simulink model "wing_landing_gear"  (R2015a)
settings: Solver=ode45  StartTime=0  StopTime=10  RelTol=1e-4  AbsTol=1e-4
model workspace (MAT data in the model file):
  grey = [0.5 0.5 0.5]
  lgrey = [0.7 0.7 0.7]
  dgrey = [0.3 0.3 0.3]
  ddgrey = [0.15 0.15 0.15]
  rho_alum = 2700
undefined symbols (not defined in the file): sigbuilder_block, X, Y, Z
libraries: sm_lib x59, sm_wing_landing_gear_lib x45, nesl_utility x7, simulink x2
(part 2 of 3)

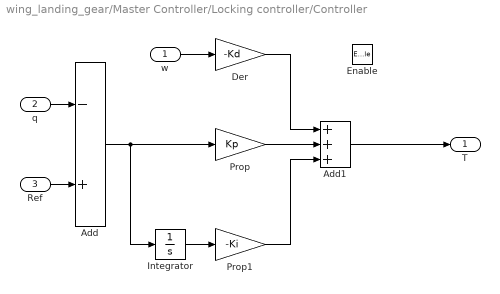
== system wing_landing_gear/Master Controller/Locking controller/Controller ==
  w : Inport
  q : Inport  Port=2
  Ref : Inport  Port=3
  Enable : EnablePort  StatesWhenEnabling=reset
  Add : Sum  Inputs=-+
  Add1 : Sum  Inputs=+++
  Der : Gain  Gain=-Kd
  Integrator : Integrator
  Prop : Gain  Gain=Kp
  Prop1 : Gain  Gain=-Ki
  T : Outport
  wires:
  Ref/1 -> Add/2
  Prop1/1 -> Add1/3
  Integrator/1 -> Prop1/1
  Add1/1 -> T/1
  Prop/1 -> Add1/2
  Der/1 -> Add1/1
  Add/1 -> Integrator/1, Prop/1
  w/1 -> Der/1
  q/1 -> Add/1

== system wing_landing_gear/Wing Landing Gear/Main Column/Actuator Cross Bar ==
  Bar A : sm_wing_landing_gear_lib/Annular Cylinder  Ro=4  Ri=1  L=25  rho=rho_alum  clr=lgrey  opc=1
  Bar B : sm_wing_landing_gear_lib/Annular Cylinder  Ro=3  Ri=1  L=5  rho=rho_alum  clr=lgrey  opc=1
  Bar C : sm_wing_landing_gear_lib/Annular Cylinder  Ro=3  Ri=1  L=5  rho=rho_alum  clr=lgrey  opc=1
  Bar D : sm_wing_landing_gear_lib/Annular Cylinder  Ro=4  Ri=1  L=15  rho=rho_alum  clr=lgrey  opc=1
  Bar E : sm_wing_landing_gear_lib/Annular Cylinder  Ro=2  Ri=0.5  L=41  rho=rho_alum  clr=lgrey  opc=1
  Reference Frame : sm_lib/Frames and Transforms/Reference Frame  BlockFunction=simmechanics.library.frames_transforms.reference_frame
  C : PMIOPort  Port=1  Side=Left
  H2 : PMIOPort  Port=2  Side=Right
  connections:
  Reference Frame/RConn1 -- Bar A/RConn1
  Bar E/LConn1 -- H2/RConn1
  Bar D/LConn1 -- Bar E/RConn1
  Bar C/LConn1 -- Bar D/RConn1
  C/RConn1 -- Bar C/RConn1 -- Bar B/LConn1
  Bar A/LConn1 -- Bar B/RConn1

== system wing_landing_gear/Wing Landing Gear/Main Column/Deploy Actuator ==
  F : Inport
  Bracket : sm_wing_landing_gear_lib/Bracket with  Circular Base  Rb=8  Tb=2  Wf=14  Tf=6  Rh=3  Oh=7  rho=rho_alum  clr=dgrey
  Bracket Transform : sm_lib/Frames and Transforms/Rigid Transform  TranslationMethod=None  TranslationLengthUnit=m  TranslationStandardAxis=+Z  TranslationStandardOffset=0  TranslationCartesianOffset=[0 0 0]  TranslationROffset=0  TranslationROffsetUnits=m  TranslationZOffset=0  TranslationZOffsetUnits=m  TranslationThetaOffset=0  TranslationThetaOffsetUnits=deg  RotationMethod=StandardAxis  RotationAngleUnits=deg  RotationStandardAxis=+X  RotationAngle=180  RotationArbitraryAxis=[0 0 1]  FollAlignAxisA=+X  BaseAlignAxisA=+Y  FollAlignAxisB=+Y  BaseAlignAxisB=+Z  RotationMatrix=[1 0 0; 0 1 0; 0 0 1]  BlockFunction=simmechanics.library.frames_transforms.rigid_transform
  Cylinder : sm_wing_landing_gear_lib/Annular Cylinder  Ro=8  Ri=7  L=45  rho=rho_alum  clr=dgrey  opc=0.5
  Cylinder Bracket Transform : sm_lib/Frames and Transforms/Rigid Transform  TranslationMethod=None  TranslationLengthUnit=m  TranslationStandardAxis=+Z  TranslationStandardOffset=0  TranslationCartesianOffset=[0 0 0]  TranslationROffset=0  TranslationROffsetUnits=m  TranslationZOffset=0  TranslationZOffsetUnits=m  TranslationThetaOffset=0  TranslationThetaOffsetUnits=deg  RotationMethod=StandardAxis  RotationAngleUnits=deg  RotationStandardAxis=+X  RotationAngle=180  RotationArbitraryAxis=[0 0 1]  FollAlignAxisA=+X  BaseAlignAxisA=+Y  FollAlignAxisB=+Y  BaseAlignAxisB=+Z  RotationMatrix=[1 0 0; 0 1 0; 0 0 1]  BlockFunction=simmechanics.library.frames_transforms.rigid_transform
  Main Piston Force : nesl_utility/Simulink-PS Converter  PhysicalDomain=network_engine_domain  SubClassName=ps_input  LeftPortType=input  RightPortType=output  PseudoPeriodic=off  Frequencies=[]  NoiseDistribution=none  NoiseParameters=[]  Unit=N  AffineConversion=off  InputFiltering=off  SimscapeFilterOrder=1  InputFilterTimeConstant=.001  UdotUserProvided=1
  Prismatic Joint1 : sm_lib/Joints/Prismatic Joint  SenseConstraintForce=off  SenseConstraintForceX=off  SenseConstraintForceY=off  SenseConstraintForceZ=off  SenseConstraintTorque=off  SenseConstraintTorqueX=off  SenseConstraintTorqueY=off  SenseConstraintTorqueZ=off  SenseTotalForce=off  SenseTotalForceX=off  SenseTotalForceY=off  SenseTotalForceZ=off  SenseTotalTorque=off  SenseTotalTorqueX=off  SenseTotalTorqueY=off  SenseTotalTorqueZ=off  CompositeWrenchDir=FollowerOnBase  CompositeWrenchFrame=BaseFrame  EquilibriumPosition=0  EquilibriumPositionUnits=cm  SpringStiffness=0  SpringStiffnessUnits=N/m  DampingCoefficient=0  DampingCoefficientUnits=N/(m/s)  TorqueActuationMode=InputTorque  MotionActuationMode=ComputedMotion  SensePosition=off  SenseVelocity=off  SenseAcceleration=off  SenseTorqueForce=off  PositionTargetSpecify=on  PositionTargetPriority=Low  PositionTargetValue=-40  PositionTargetValueUnits=cm  VelocityTargetSpecify=off  VelocityTargetPriority=High  VelocityTargetValue=0  VelocityTargetValueUnits=m/s  BlockFunction=simmechanics.library.joints.prismatic_joint
  Retraction Piston : Subsystem  mask(Piston with Bracket){Rb=7, Th=2, Rp=5, Lp=41, Wf=10, Tf=3, Oh=8, Rh=3, rho=rho_alum, clr=grey}
      mask prompts: Rb "Bore radius (cm)"; Th "Piston head thickness (cm)"; Rp "Piston radius (cm)"; Lp "Piston length (cm)"; Wf "Bracket width (cm)"; Tf "Bracket thickness (cm)"; Oh "Hole offset (cm)"; Rh "Hole radius (cm)"; rho "Density (kg/m^3)"; clr "Color"
      mask init:
      | flange_lower_sec = [Wf/2 0; Wf/2 Oh];
      | theta = (0:-1:-180)*pi/180;
      | x = Rh*cos(theta');
      | y = Oh + Rh*sin(theta');
      | flange_lower_sec = [flange_lower_sec; [x y]];
      | flange_lower_sec = [flange_lower_sec; -Wf/2 Oh; -Wf/2 0];
      | 
      | theta = (0:1:180)*pi/180;
      | x = (Wf/2)*cos(theta');
      | y = (Wf/2)*sin(theta');
      | flange_upper_sec = [x y];
      | theta = (180:-1:0)*pi/180;
      | x = Rh*cos(theta');
      | y = Rh*sin(theta');
      | flange_upper_sec = [flange_upper_sec; [x y]];
      | 
      | Tb = 2;
      | Lpr = Lp - Tb;
      mask Display:
      | image(imread('sm_wlandgear_piston.png'));
      | port_label('LConn',1,'H');
      | port_label('RConn',1,'B');
  C : PMIOPort  Port=1  Side=Left
  P : PMIOPort  Port=2  Side=Right
  wires:
  F/1 -> Main Piston Force/1
  connections:
  Bracket/RConn1 -- Bracket Transform/LConn1
  Bracket Transform/RConn1 -- C/RConn1
  Cylinder Bracket Transform/RConn1 -- Bracket/LConn1
  Cylinder Bracket Transform/LConn1 -- Cylinder/LConn1
  Prismatic Joint1/LConn1 -- Cylinder/RConn1
  Retraction Piston/RConn1 -- Prismatic Joint1/RConn1
  P/RConn1 -- Retraction Piston/LConn1
  Prismatic Joint1/LConn2 -- Main Piston Force/RConn1

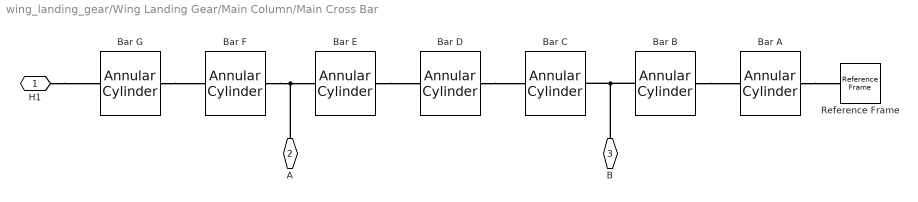
== system wing_landing_gear/Wing Landing Gear/Main Column/Main Cross Bar ==
  Bar A : sm_wing_landing_gear_lib/Annular Cylinder  Ro=7  Ri=2  L=25  rho=rho_alum  clr=lgrey  opc=1
  Bar B : sm_wing_landing_gear_lib/Annular Cylinder  Ro=5  Ri=2  L=5  rho=rho_alum  clr=lgrey  opc=1
  Bar C : sm_wing_landing_gear_lib/Annular Cylinder  Ro=5  Ri=2  L=5  rho=rho_alum  clr=lgrey  opc=1
  Bar D : sm_wing_landing_gear_lib/Annular Cylinder  Ro=7  Ri=2  L=33  rho=rho_alum  clr=lgrey  opc=1
  Bar E : sm_wing_landing_gear_lib/Annular Cylinder  Ro=3  Ri=2  L=4  rho=rho_alum  clr=lgrey  opc=1
  Bar F : sm_wing_landing_gear_lib/Annular Cylinder  Ro=3  Ri=2  L=4  rho=rho_alum  clr=lgrey  opc=1
  Bar G : sm_wing_landing_gear_lib/Annular Cylinder  Ro=7  Ri=2  L=15  rho=rho_alum  clr=lgrey  opc=1
  Reference Frame : sm_lib/Frames and Transforms/Reference Frame  BlockFunction=simmechanics.library.frames_transforms.reference_frame
  H1 : PMIOPort  Port=1  Side=Left
  A : PMIOPort  Port=2  Side=Right
  B : PMIOPort  Port=3  Side=Right
  connections:
  B/RConn1 -- Bar C/RConn1 -- Bar B/LConn1
  A/RConn1 -- Bar E/LConn1 -- Bar F/RConn1
  H1/RConn1 -- Bar G/LConn1
  Bar B/RConn1 -- Bar A/LConn1
  Bar D/RConn1 -- Bar C/LConn1
  Bar E/RConn1 -- Bar D/LConn1
  Bar G/RConn1 -- Bar F/LConn1
  Bar A/RConn1 -- Reference Frame/RConn1

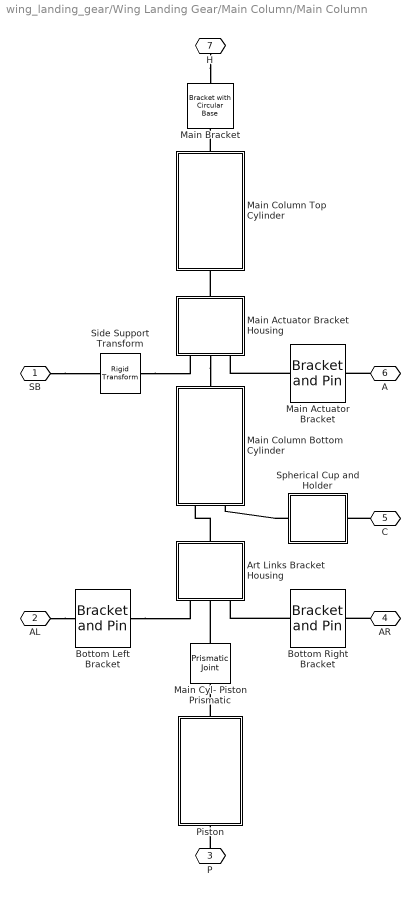
== system wing_landing_gear/Wing Landing Gear/Main Column/Main Column ==
  Art Links Bracket Housing : Subsystem  mask(Bracket Housing){Ro=12, Ri=8, L=12, rho=rho_alum, clr=dgrey}
      mask prompts: Ro "Cylinder outer radius (cm)"; Ri "Cylinder inner radius (cm)"; L "Cylinder length (cm)"; rho "Density (kg/m^3)"; clr "Color"
      mask help: This part holds the brackets that connect to the articulating links. The Dimensions can be specified below.
      mask init:
      | theta = (180:-1:0)*pi/180;
      | t_semi_annular_sec = [Ri*cos(theta') Ri*sin(theta')];
      | theta = (0:1:180)*pi/180;
      | t_semi_annular_sec = [t_semi_annular_sec; Ro*cos(theta') Ro*sin(theta')];
      | b_semi_annular_sec = [t_semi_annular_sec(end:-1:1,1) -t_semi_annular_sec(end:-1:1,2)];
      mask Display:
      | image(imread('sm_wlandgear_bhousing.png'));
      | port_label('LConn',1,'L')
      | port_label('LConn',2,'B')
      | port_label('LConn',3,'R')
      | port_label('RConn',1,'T')
  Bottom Left Bracket : sm_wing_landing_gear_lib/Bracket and Pin  Wb=6  Tb=2  L=12  Rb=12  Ro=4  Wf=5  Ri=2  Lp=14  rho=1000  clr=[0.3 0.3 0.3]
  Bottom Right Bracket : sm_wing_landing_gear_lib/Bracket and Pin  Wb=6  Tb=2  L=12  Rb=12  Ro=4  Wf=5  Ri=2  Lp=14  rho=1000  clr=[0.3 0.3 0.3]
  Main Bracket : sm_wing_landing_gear_lib/Bracket with  Circular Base  Rb=12  Tb=6  Wf=22  Tf=6  Rh=5  Oh=9  rho=rho_alum  clr=dgrey
  Main Actuator Bracket Housing : Subsystem  mask(Bracket Housing){Ro=12, Ri=8, L=20, rho=rho_alum, clr=dgrey}
      mask prompts: Ro "Cylinder outer radius (cm)"; Ri "Cylinder inner radius (cm)"; L "Cylinder length (cm)"; rho "Density (kg/m^3)"; clr "Color"
      mask help: This part holds the brackets that connect to the articulating links. The Dimensions can be specified below.
      mask init: same as wing_landing_gear/Wing Landing Gear/Main Column/Main Column/Art Links Bracket Housing
      mask Display:
      | image(imread('sm_wlandgear_bhousing.png'));
      | port_label('LConn',1,'L')
      | port_label('LConn',2,'B')
      | port_label('LConn',3,'R')
      | port_label('RConn',1,'T')
  Main Actuator Bracket : sm_wing_landing_gear_lib/Bracket and Pin  Wb=9  Tb=2  L=20  Rb=12  Ro=7  Wf=12  Ri=3  Lp=14  rho=1000  clr=[0.3 0.3 0.3]
  Main Column Bottom Cylinder : Subsystem  mask(Main Column Bottom Cylinder){Ro=12, Ri=8, L=45, Oh=2.5, Ah=0, rho=rho_alum, clr=lgrey}
      mask prompts: Ro "Cylinder outer radius (cm)"; Ri "Cylinder inner radius (cm)"; L "Cylinder length (cm)"; Oh "Spherical joint holder offset from base (cm)"; Ah "Spherical joint holder angle (deg)"; rho "Density (kg/m^3)"; clr "Color"
      mask init: same as wing_landing_gear/Wing Landing Gear/Main Column/Main Column/Art Links Bracket Housing
      mask Display:
      | image(imread('sm_wlandgear_botcyl.png'));
      | port_label('Rconn',1,'T')
      | port_label('Lconn',1,'B')
      | port_label('Lconn',2,'S')
  Main Column Top Cylinder : Subsystem  mask(Main Column Bottom Cylinder){Ro=12, Ri=8, L=60, rho=rho_alum, clr=lgrey}
      mask prompts: Ro "Cylinder outer radius (cm)"; Ri "Cylinder inner radius (cm)"; L "Cylinder length (cm)"; rho "Density (kg/m^3)"; clr "Color"
      mask init: same as wing_landing_gear/Wing Landing Gear/Main Column/Main Column/Art Links Bracket Housing
      mask Display:
      | image(imread('sm_wlandgear_botcyl.png'));
      | port_label('Rconn',1,'T')
      | port_label('Lconn',1,'B')
  Main Cyl- Piston Prismatic : sm_lib/Joints/Prismatic Joint  SenseConstraintForce=off  SenseConstraintForceX=off  SenseConstraintForceY=off  SenseConstraintForceZ=off  SenseConstraintTorque=off  SenseConstraintTorqueX=off  SenseConstraintTorqueY=off  SenseConstraintTorqueZ=off  SenseTotalForce=off  SenseTotalForceX=off  SenseTotalForceY=off  SenseTotalForceZ=off  SenseTotalTorque=off  SenseTotalTorqueX=off  SenseTotalTorqueY=off  SenseTotalTorqueZ=off  CompositeWrenchDir=FollowerOnBase  CompositeWrenchFrame=BaseFrame  EquilibriumPosition=30  EquilibriumPositionUnits=cm  SpringStiffness=250000  SpringStiffnessUnits=N/m  DampingCoefficient=50000  DampingCoefficientUnits=N/(m/s)  TorqueActuationMode=NoTorque  MotionActuationMode=ComputedMotion  SensePosition=off  SenseVelocity=off  SenseAcceleration=off  SenseTorqueForce=off  PositionTargetSpecify=on  PositionTargetPriority=Low  PositionTargetValue=30  PositionTargetValueUnits=cm  VelocityTargetSpecify=off  VelocityTargetPriority=Low  VelocityTargetValue=0  VelocityTargetValueUnits=m/s  BlockFunction=simmechanics.library.joints.prismatic_joint
  "Piston " : Subsystem  mask(Main Column Piston){Ro=8, Ri=4, L=55, Rf=12, Tf=1.5, rho=rho_alum, clr=lgrey}
      mask prompts: Ro "Cylinder outer radius (cm)"; Ri "Cylinder inner radius (cm)"; L "Cylinder length (cm)"; Rf "Flange outer radius (cm)"; Tf "Flange thickness (cm)"; rho "Density (kg/m^3)"; clr "Color"
      mask help: This is the Piston of the main column. The dimensions of the Piston can be specified below.
      mask init: same as wing_landing_gear/Wing Landing Gear/Main Column/Main Column/Art Links Bracket Housing
      mask Display: image(imread('sm_wlandgear_mainpiston.png'));
  Side Support Transform : sm_lib/Frames and Transforms/Rigid Transform  TranslationMethod=Cartesian  TranslationLengthUnit=cm  TranslationStandardAxis=-Y  TranslationStandardOffset=0  TranslationCartesianOffset=[-12 -12 0]  TranslationROffset=0  TranslationROffsetUnits=cm  TranslationZOffset=0  TranslationZOffsetUnits=cm  TranslationThetaOffset=0  TranslationThetaOffsetUnits=deg  RotationMethod=StandardAxis  RotationAngleUnits=deg  RotationStandardAxis=-Z  RotationAngle=180  RotationArbitraryAxis=[0 0 1]  FollAlignAxisA=+X  BaseAlignAxisA=-X  FollAlignAxisB=+Y  BaseAlignAxisB=-Y  RotationMatrix=[1 0 0; 0 1 0; 0 0 1]  BlockFunction=simmechanics.library.frames_transforms.rigid_transform
  Spherical Cup and Holder : Subsystem  mask(Spherical Cup and Holder){Wb=20, Rb=12, Ro=6, Hh=8, Rci=4, Rco=6, Oh=12, rho=rho_alum, cclr=lgrey, hclr=dgrey}
      mask prompts: Wb "Base width (cm)"; Rb "Radius of curvature (base face) (cm)"; Ro "Radius of curvature (outer face) (cm)"; Hh "Thickness (cm)"; Rci "Cup inner radius (cm)"; Rco "Cup outer radius (cm)"; Oh "Cup offset (cm)"; rho "Density (kg/m^3)"; cclr "Cup color"; hclr "Holder color"
      mask init:
      | Hp = sqrt((Wb/2)^2 + Oh^2);
      | th = acos(Oh/Hp) + acos(Ro/Hp);
      | theta = linspace(th-pi,0,25);
      | hinge_sec_a = [Oh+Ro*cos(theta') Ro*sin(theta')];
      | 
      | th = asin(Wb/(2*Rb));
      | theta = linspace(0,-th,50);  
      | hinge_sec_a = [hinge_sec_a;
      |              Rb*cos(theta')-Rb Rb*sin(theta')];
      | 
      | hinge_sec_b = flipud([hinge_sec_a(:,1) -hinge_sec_a(:,2)]);
      mask Display:
      | image(imread('sm_wlandgear_cupholder.png'));
      | port_label('LConn',1,'B');
      | port_label('RConn',1,'C');
  SB : PMIOPort  Port=1  Side=Right
  AL : PMIOPort  Port=2  Side=Right
  P : PMIOPort  Port=3  Side=Right
  AR : PMIOPort  Port=4  Side=Right
  C : PMIOPort  Port=5  Side=Right
  A : PMIOPort  Port=6  Side=Right
  H : PMIOPort  Port=7  Side=Left
  connections:
  SB/RConn1 -- Side Support Transform/RConn1
  Side Support Transform/LConn1 -- Main Actuator Bracket Housing/LConn1
  P/RConn1 -- "Piston "/RConn1
  AR/RConn1 -- Bottom Right Bracket/RConn1
  AL/RConn1 -- Bottom Left Bracket/RConn1
  C/RConn1 -- Spherical Cup and Holder/RConn1
  A/RConn1 -- Main Actuator Bracket/RConn1
  H/RConn1 -- Main Bracket/RConn1
  "Piston "/LConn1 -- Main Cyl- Piston Prismatic/RConn1
  Main Column Top Cylinder/RConn1 -- Main Bracket/LConn1
  Spherical Cup and Holder/LConn1 -- Main Column Bottom Cylinder/LConn2
  Main Actuator Bracket Housing/RConn1 -- Main Column Top Cylinder/LConn1
  Main Actuator Bracket/LConn1 -- Main Actuator Bracket Housing/LConn3
  Main Actuator Bracket Housing/LConn2 -- Main Column Bottom Cylinder/RConn1
  Art Links Bracket Housing/RConn1 -- Main Column Bottom Cylinder/LConn1
  Main Cyl- Piston Prismatic/LConn1 -- Art Links Bracket Housing/LConn2
  Bottom Right Bracket/LConn1 -- Art Links Bracket Housing/LConn3
  Bottom Left Bracket/LConn1 -- Art Links Bracket Housing/LConn1

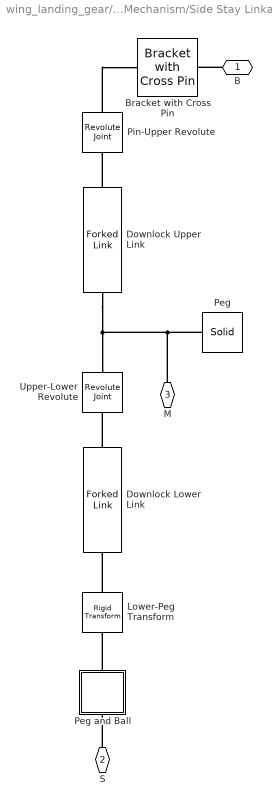
== system wing_landing_gear/Wing Landing Gear/Main Column Locking Mechanism/Side Stay Linkage ==
  Bracket with Cross Pin : sm_wing_landing_gear_lib/Bracket with Cross Pin  Lb=14  Tb=3  Gb=5  Ro=7  Ri=4  Oh=14  Rp=4  Lh=40  Ohp=10  Lv=20  Ov=10  rho=rho_alum  bclr=dgrey  pclr=lgrey
  Downlock Lower Link : sm_wing_landing_gear_lib/Forked Link  L1=111  L2=20  L3=7  L4=15  L5=10  L6=4  H1=16  H2=10  H3=1  H4=5  T=12  rho=rho_alum  clr=dgrey
  Downlock Upper Link : sm_wing_landing_gear_lib/Forked Link  L1=110.5  L2=20  L3=11  L4=15  L5=10  L6=4  H1=16  H2=10  H3=1  H4=5  T=12  rho=rho_alum  clr=dgrey
  Lower-Peg Transform : sm_lib/Frames and Transforms/Rigid Transform  TranslationMethod=StandardAxis  TranslationLengthUnit=cm  TranslationStandardAxis=+X  TranslationStandardOffset=6  TranslationCartesianOffset=[0 0 0]  TranslationROffset=0  TranslationROffsetUnits=m  TranslationZOffset=0  TranslationZOffsetUnits=m  TranslationThetaOffset=0  TranslationThetaOffsetUnits=deg  RotationMethod=AlignedAxes  RotationAngleUnits=deg  RotationStandardAxis=+Z  RotationAngle=0  RotationArbitraryAxis=[0 0 1]  FollAlignAxisA=+Z  BaseAlignAxisA=+X  FollAlignAxisB=+X  BaseAlignAxisB=-Z  RotationMatrix=[1 0 0; 0 1 0; 0 0 1]  BlockFunction=simmechanics.library.frames_transforms.rigid_transform
  Peg : sm_lib/Body Elements/Solid  InertiaType=CalculateFromGeometry  Mass=1  MassUnits=kg  CenterOfMass=[0 0 0]  CenterOfMassUnits=m  MomentsOfInertia=[1 1 1]  MomentsOfInertiaUnits=kg*m^2  ProductsOfInertia=[0 0 0]  ProductsOfInertiaUnits=kg*m^2  DensityBased=on  Density=rho_alum  DensityUnits=kg/(m^3)  GraphicType=FromGeometry  MarkerShape=Sphere  MarkerSize=10  MarkerSizeUnits=m  GraphicVisPropType=SimpleVisualProperties  GraphicDiffuseColor=lgrey  GraphicSpecularColor=[0.5 0.5 0.5 1.0]  GraphicAmbientColor=[0.5 0.0 0.0 1.0]  GraphicEmissiveColor=[0.0 0.0 0.0 1.0]  GraphicShininess=75  GraphicOpacity=1.0  GeometryShape=Cylinder  RectangleSize=[1 1]  RectangleSizeUnits=m  BrickDimensions=[1 1 1]  BrickDimensionUnits=m  CylinderRadius=4  CylinderRadiusUnits=cm  CylinderLength=22  CylinderLengthUnits=cm  SphereRadius=1  SphereRadiusUnits=m  EllipsoidRadii=[1 1 1]  EllipsoidRadiiUnits=m  ExtrusionCrossSection=[1 1; -1 1; -1 -1; 1 -1]  ExtrusionCrossSectionUnits=m  ExtrusionLength=1  ExtrusionLengthUnits=m  PolygonNumSides=3  PolygonOuterRadius=1  PolygonOuterRadiusUnits=m  ExtGeomFileType=STL  ExtGeomFileUnits=m  RevolutionCrossSection=[1 1; 1 -1; 2 -1; 2 1]  RevolutionCrossSectionUnits=m  RevolutionExtent=Full  RevolutionAngle=180  RevolutionAngleUnits=deg  BlockFunction=simmechanics.library.body_elements.solid
  Peg and Ball : Subsystem  mask{Lp=5, Rp=2, Rb=4, rho=rho_alum, clr=lgrey}
      mask prompts: Lp "Length of peg (cm)"; Rp "Radius of peg (cm)"; Rb "Radius of ball (cm)"; rho "Density (kg/m^3)"; clr "Color"
  Pin-Upper Revolute : sm_lib/Joints/Revolute Joint  SenseConstraintForce=off  SenseConstraintForceX=off  SenseConstraintForceY=off  SenseConstraintForceZ=off  SenseConstraintTorque=off  SenseConstraintTorqueX=off  SenseConstraintTorqueY=off  SenseConstraintTorqueZ=off  SenseTotalForce=off  SenseTotalForceX=off  SenseTotalForceY=off  SenseTotalForceZ=off  SenseTotalTorque=off  SenseTotalTorqueX=off  SenseTotalTorqueY=off  SenseTotalTorqueZ=off  CompositeWrenchDir=FollowerOnBase  CompositeWrenchFrame=BaseFrame  EquilibriumPosition=0  EquilibriumPositionUnits=rad  SpringStiffness=0  SpringStiffnessUnits=N*m/rad  DampingCoefficient=0  DampingCoefficientUnits=N*m/(rad/s)  TorqueActuationMode=NoTorque  MotionActuationMode=ComputedMotion  SensePosition=off  SenseVelocity=off  SenseAcceleration=off  SenseTorqueForce=off  PositionTargetSpecify=on  PositionTargetPriority=Low  PositionTargetValue=-90  PositionTargetValueUnits=deg  VelocityTargetSpecify=off  VelocityTargetPriority=Low  VelocityTargetValue=0  VelocityTargetValueUnits=rad/s  BlockFunction=simmechanics.library.joints.revolute_joint
  Upper-Lower Revolute : sm_lib/Joints/Revolute Joint  SenseConstraintForce=off  SenseConstraintForceX=off  SenseConstraintForceY=off  SenseConstraintForceZ=off  SenseConstraintTorque=off  SenseConstraintTorqueX=off  SenseConstraintTorqueY=off  SenseConstraintTorqueZ=off  SenseTotalForce=off  SenseTotalForceX=off  SenseTotalForceY=off  SenseTotalForceZ=off  SenseTotalTorque=off  SenseTotalTorqueX=off  SenseTotalTorqueY=off  SenseTotalTorqueZ=off  CompositeWrenchDir=FollowerOnBase  CompositeWrenchFrame=BaseFrame  EquilibriumPosition=0  EquilibriumPositionUnits=rad  SpringStiffness=0  SpringStiffnessUnits=N*m/rad  DampingCoefficient=0  DampingCoefficientUnits=N*m/(rad/s)  TorqueActuationMode=NoTorque  MotionActuationMode=ComputedMotion  SensePosition=off  SenseVelocity=off  SenseAcceleration=off  SenseTorqueForce=off  PositionTargetSpecify=on  PositionTargetPriority=Low  PositionTargetValue=-150  PositionTargetValueUnits=deg  VelocityTargetSpecify=off  VelocityTargetPriority=Low  VelocityTargetValue=0  VelocityTargetValueUnits=rad/s  BlockFunction=simmechanics.library.joints.revolute_joint
  B : PMIOPort  Port=1  Side=Left
  S : PMIOPort  Port=2  Side=Right
  M : PMIOPort  Port=3  Side=Right
  connections:
  Peg and Ball/LConn1 -- Lower-Peg Transform/RConn1
  Lower-Peg Transform/LConn1 -- Downlock Lower Link/RConn1
  S/RConn1 -- Peg and Ball/RConn1
  Downlock Lower Link/LConn1 -- Upper-Lower Revolute/RConn1
  Peg/RConn1 -- Upper-Lower Revolute/LConn1 -- Downlock Upper Link/RConn1 -- M/RConn1
  Downlock Upper Link/LConn1 -- Pin-Upper Revolute/RConn1
  B/RConn1 -- Bracket with Cross Pin/RConn1
  Pin-Upper Revolute/LConn1 -- Bracket with Cross Pin/LConn1

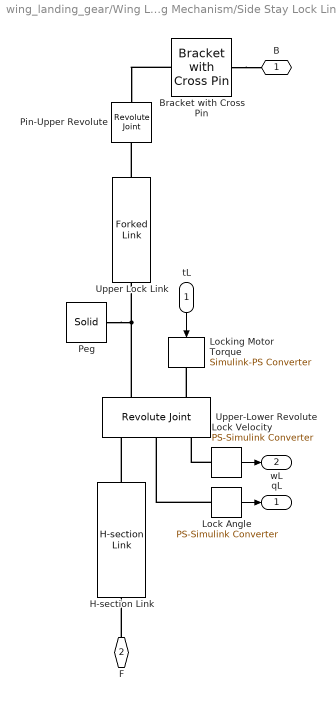
== system wing_landing_gear/Wing Landing Gear/Main Column Locking Mechanism/Side Stay Lock Linkage ==
  tL : Inport
  Bracket with Cross Pin : sm_wing_landing_gear_lib/Bracket with Cross Pin  Lb=14  Tb=3  Gb=5  Ro=7  Ri=4  Oh=14  Rp=4  Lh=40  Ohp=10  Lv=20  Ov=10  rho=rho_alum  bclr=dgrey  pclr=lgrey
  H-section Link : sm_wing_landing_gear_lib/H-section Link  Lb=5  Wb=22  Tb=12  Tf=3  Oh=25.5  Ri=4  rho=rho_alum  clr=dgrey
  Lock Angle : nesl_utility/PS-Simulink Converter  PhysicalDomain=network_engine_domain  SubClassName=ps_output  LeftPortType=input  RightPortType=output  PseudoPeriodic=off  Frequencies=[]  Unit=deg  AffineConversion=off
  Lock Velocity : nesl_utility/PS-Simulink Converter  PhysicalDomain=network_engine_domain  SubClassName=ps_output  LeftPortType=input  RightPortType=output  PseudoPeriodic=off  Frequencies=[]  Unit=deg/s  AffineConversion=off
  Locking Motor Torque : nesl_utility/Simulink-PS Converter  PhysicalDomain=network_engine_domain  SubClassName=ps_input  LeftPortType=input  RightPortType=output  PseudoPeriodic=off  Frequencies=[]  NoiseDistribution=none  NoiseParameters=[]  Unit=N*m  AffineConversion=off  InputFiltering=off  SimscapeFilterOrder=1  InputFilterTimeConstant=.001  UdotUserProvided=1
  Peg : sm_lib/Body Elements/Solid  InertiaType=CalculateFromGeometry  Mass=1  MassUnits=kg  CenterOfMass=[0 0 0]  CenterOfMassUnits=m  MomentsOfInertia=[1 1 1]  MomentsOfInertiaUnits=kg*m^2  ProductsOfInertia=[0 0 0]  ProductsOfInertiaUnits=kg*m^2  DensityBased=on  Density=rho_alum  DensityUnits=kg/(m^3)  GraphicType=FromGeometry  MarkerShape=Sphere  MarkerSize=10  MarkerSizeUnits=m  GraphicVisPropType=SimpleVisualProperties  GraphicDiffuseColor=lgrey  GraphicSpecularColor=[0.5 0.5 0.5 1.0]  GraphicAmbientColor=[0.5 0.0 0.0 1.0]  GraphicEmissiveColor=[0.0 0.0 0.0 1.0]  GraphicShininess=75  GraphicOpacity=1.0  GeometryShape=Cylinder  RectangleSize=[1 1]  RectangleSizeUnits=m  BrickDimensions=[1 1 1]  BrickDimensionUnits=m  CylinderRadius=4  CylinderRadiusUnits=cm  CylinderLength=22  CylinderLengthUnits=cm  SphereRadius=1  SphereRadiusUnits=m  EllipsoidRadii=[1 1 1]  EllipsoidRadiiUnits=m  ExtrusionCrossSection=[1 1; -1 1; -1 -1; 1 -1]  ExtrusionCrossSectionUnits=m  ExtrusionLength=1  ExtrusionLengthUnits=m  PolygonNumSides=3  PolygonOuterRadius=1  PolygonOuterRadiusUnits=m  ExtGeomFileType=STL  ExtGeomFileUnits=m  RevolutionCrossSection=[1 1; 1 -1; 2 -1; 2 1]  RevolutionCrossSectionUnits=m  RevolutionExtent=Full  RevolutionAngle=180  RevolutionAngleUnits=deg  BlockFunction=simmechanics.library.body_elements.solid
  Pin-Upper Revolute : sm_lib/Joints/Revolute Joint  SenseConstraintForce=off  SenseConstraintForceX=off  SenseConstraintForceY=off  SenseConstraintForceZ=off  SenseConstraintTorque=off  SenseConstraintTorqueX=off  SenseConstraintTorqueY=off  SenseConstraintTorqueZ=off  SenseTotalForce=off  SenseTotalForceX=off  SenseTotalForceY=off  SenseTotalForceZ=off  SenseTotalTorque=off  SenseTotalTorqueX=off  SenseTotalTorqueY=off  SenseTotalTorqueZ=off  CompositeWrenchDir=FollowerOnBase  CompositeWrenchFrame=BaseFrame  EquilibriumPosition=0  EquilibriumPositionUnits=rad  SpringStiffness=0  SpringStiffnessUnits=N*m/rad  DampingCoefficient=0  DampingCoefficientUnits=N*m/(rad/s)  TorqueActuationMode=NoTorque  MotionActuationMode=ComputedMotion  SensePosition=off  SenseVelocity=off  SenseAcceleration=off  SenseTorqueForce=off  PositionTargetSpecify=off  PositionTargetPriority=Low  PositionTargetValue=-90  PositionTargetValueUnits=deg  VelocityTargetSpecify=off  VelocityTargetPriority=Low  VelocityTargetValue=0  VelocityTargetValueUnits=rad/s  BlockFunction=simmechanics.library.joints.revolute_joint
  Upper Lock Link : sm_wing_landing_gear_lib/Forked Link  L1=72.5  L2=20  L3=11  L4=15  L5=10  L6=4  H1=16  H2=10  H3=1  H4=5  T=11  rho=rho_alum  clr=dgrey
  Upper-Lower Revolute : sm_lib/Joints/Revolute Joint  SenseConstraintForce=off  SenseConstraintForceX=off  SenseConstraintForceY=off  SenseConstraintForceZ=off  SenseConstraintTorque=off  SenseConstraintTorqueX=off  SenseConstraintTorqueY=off  SenseConstraintTorqueZ=off  SenseTotalForce=off  SenseTotalForceX=off  SenseTotalForceY=off  SenseTotalForceZ=off  SenseTotalTorque=off  SenseTotalTorqueX=off  SenseTotalTorqueY=off  SenseTotalTorqueZ=off  CompositeWrenchDir=FollowerOnBase  CompositeWrenchFrame=BaseFrame  EquilibriumPosition=0  EquilibriumPositionUnits=rad  SpringStiffness=0  SpringStiffnessUnits=N*m/rad  DampingCoefficient=0  DampingCoefficientUnits=N*m/(rad/s)  TorqueActuationMode=InputTorque  MotionActuationMode=ComputedMotion  SensePosition=on  SenseVelocity=on  SenseAcceleration=off  SenseTorqueForce=off  PositionTargetSpecify=on  PositionTargetPriority=Low  PositionTargetValue=20  PositionTargetValueUnits=deg  VelocityTargetSpecify=off  VelocityTargetPriority=Low  VelocityTargetValue=0  VelocityTargetValueUnits=rad/s  BlockFunction=simmechanics.library.joints.revolute_joint
  B : PMIOPort  Port=1  Side=Left
  F : PMIOPort  Port=2  Side=Right
  qL : Outport
  wL : Outport  Port=2
  wires:
  tL/1 -> Locking Motor Torque/1
  Lock Velocity/1 -> wL/1
  Lock Angle/1 -> qL/1
  connections:
  F/RConn1 -- H-section Link/LConn1
  H-section Link/RConn1 -- Upper-Lower Revolute/RConn1
  Peg/RConn1 -- Upper Lock Link/RConn1 -- Upper-Lower Revolute/LConn1
  Upper Lock Link/LConn1 -- Pin-Upper Revolute/RConn1
  Bracket with Cross Pin/LConn1 -- Pin-Upper Revolute/LConn1
  Bracket with Cross Pin/RConn1 -- B/RConn1
  Upper-Lower Revolute/LConn2 -- Locking Motor Torque/RConn1
  Lock Velocity/LConn1 -- Upper-Lower Revolute/RConn3
  Lock Angle/LConn1 -- Upper-Lower Revolute/RConn2

== system wing_landing_gear/Master Controller/Control Coordinator/Ref Signal/If Action Subsystem ==
  qM : Inport
  Action Port : ActionPort  ActionType=then
  Abs : Abs
  Compare To Constant1 : simulink/Logic and Bit Operations/Compare To Constant  relop=<=  const=On_act_ang  OutDataTypeStr=boolean
  Constant : Constant  Value=lock_tgt
  R : Outport  OutDataTypeStr=double  InitialOutput=lock_tgt*pi/180
  En : Outport  Port=2  OutDataTypeStr=boolean  InitialOutput=false
  wires:
  Compare To Constant1/1 -> En/1
  Constant/1 -> R/1
  qM/1 -> Abs/1
  Abs/1 -> Compare To Constant1/1

== system wing_landing_gear/Master Controller/Control Coordinator/Ref Signal/If Action Subsystem1 ==
  qM : Inport
  Action Port : ActionPort  ActionType=else
  Abs : Abs
  Compare To Constant1 : simulink/Logic and Bit Operations/Compare To Constant  relop=<=  const=Off_act_ang  OutDataTypeStr=boolean
  Constant : Constant  Value=unlock_tgt
  R : Outport  OutDataTypeStr=double  InitialOutput=lock_tgt*pi/180
  En : Outport  Port=2  OutDataTypeStr=boolean  InitialOutput=true
  wires:
  Compare To Constant1/1 -> En/1
  Constant/1 -> R/1
  qM/1 -> Abs/1
  Abs/1 -> Compare To Constant1/1

== system wing_landing_gear/Wing Landing Gear/Main Column/Deploy Actuator/Retraction Piston ==
  Base Transform : sm_lib/Frames and Transforms/Rigid Transform  TranslationMethod=StandardAxis  TranslationLengthUnit=cm  TranslationStandardAxis=-Z  TranslationStandardOffset=(Lpr+Th)/2  TranslationCartesianOffset=[0 0 0]  TranslationROffset=0  TranslationROffsetUnits=m  TranslationZOffset=0  TranslationZOffsetUnits=m  TranslationThetaOffset=0  TranslationThetaOffsetUnits=deg  RotationMethod=None  RotationAngleUnits=deg  RotationStandardAxis=+Z  RotationAngle=0  RotationArbitraryAxis=[0 0 1]  FollAlignAxisA=+X  BaseAlignAxisA=-X  FollAlignAxisB=+Y  BaseAlignAxisB=-Y  RotationMatrix=[1 0 0; 0 1 0; 0 0 1]  BlockFunction=simmechanics.library.frames_transforms.rigid_transform
  Bracket : sm_wing_landing_gear_lib/Bracket with  Circular Base  Rb=Rp  Tb=2  Wf=Wf  Tf=Tf  Rh=Rh  Oh=Oh  rho=rho  clr=clr
  Flange Transform : sm_lib/Frames and Transforms/Rigid Transform  TranslationMethod=StandardAxis  TranslationLengthUnit=cm  TranslationStandardAxis=+Z  TranslationStandardOffset=Lpr/2  TranslationCartesianOffset=[0 0 0]  TranslationROffset=0  TranslationROffsetUnits=m  TranslationZOffset=0  TranslationZOffsetUnits=m  TranslationThetaOffset=0  TranslationThetaOffsetUnits=deg  RotationMethod=None  RotationAngleUnits=deg  RotationStandardAxis=+Z  RotationAngle=0  RotationArbitraryAxis=[0 0 1]  FollAlignAxisA=+Z  BaseAlignAxisA=-Y  FollAlignAxisB=+Y  BaseAlignAxisB=+Z  RotationMatrix=[1 0 0; 0 1 0; 0 0 1]  BlockFunction=simmechanics.library.frames_transforms.rigid_transform
  Piston Head : sm_lib/Body Elements/Solid  InertiaType=CalculateFromGeometry  Mass=1  MassUnits=kg  CenterOfMass=[0 0 0]  CenterOfMassUnits=m  MomentsOfInertia=[1 1 1]  MomentsOfInertiaUnits=kg*m^2  ProductsOfInertia=[0 0 0]  ProductsOfInertiaUnits=kg*m^2  DensityBased=on  Density=rho  DensityUnits=kg/(m^3)  GraphicType=FromGeometry  MarkerShape=Sphere  MarkerSize=10  MarkerSizeUnits=m  GraphicVisPropType=SimpleVisualProperties  GraphicDiffuseColor=clr  GraphicSpecularColor=[0.5 0.5 0.5 1.0]  GraphicAmbientColor=[0.5 0.0 0.0 1.0]  GraphicEmissiveColor=[0.0 0.0 0.0 1.0]  GraphicShininess=75  GraphicOpacity=1.0  GeometryShape=Cylinder  RectangleSize=[1 1]  RectangleSizeUnits=m  BrickDimensions=[1 1 1]  BrickDimensionUnits=m  CylinderRadius=Rb  CylinderRadiusUnits=cm  CylinderLength=Th  CylinderLengthUnits=cm  SphereRadius=1  SphereRadiusUnits=m  EllipsoidRadii=[1 1 1]  EllipsoidRadiiUnits=m  ExtrusionCrossSection=[1 1; -1 1; -1 -1; 1 -1]  ExtrusionCrossSectionUnits=m  ExtrusionLength=1  ExtrusionLengthUnits=m  PolygonNumSides=3  PolygonOuterRadius=1  PolygonOuterRadiusUnits=m  ExtGeomFileType=STL  ExtGeomFileUnits=m  RevolutionCrossSection=[1 1; 1 -1; 2 -1; 2 1]  RevolutionCrossSectionUnits=m  RevolutionExtent=Full  RevolutionAngle=180  RevolutionAngleUnits=deg  BlockFunction=simmechanics.library.body_elements.solid
  Piston Rod : sm_lib/Body Elements/Solid  InertiaType=CalculateFromGeometry  Mass=1  MassUnits=kg  CenterOfMass=[0 0 0]  CenterOfMassUnits=m  MomentsOfInertia=[1 1 1]  MomentsOfInertiaUnits=kg*m^2  ProductsOfInertia=[0 0 0]  ProductsOfInertiaUnits=kg*m^2  DensityBased=on  Density=rho  DensityUnits=kg/(m^3)  GraphicType=FromGeometry  MarkerShape=Sphere  MarkerSize=10  MarkerSizeUnits=m  GraphicVisPropType=SimpleVisualProperties  GraphicDiffuseColor=clr  GraphicSpecularColor=[0.5 0.5 0.5 1.0]  GraphicAmbientColor=[0.5 0.0 0.0 1.0]  GraphicEmissiveColor=[0.0 0.0 0.0 1.0]  GraphicShininess=75  GraphicOpacity=1.0  GeometryShape=Cylinder  RectangleSize=[1 1]  RectangleSizeUnits=m  BrickDimensions=[1 1 1]  BrickDimensionUnits=m  CylinderRadius=Rp  CylinderRadiusUnits=cm  CylinderLength=Lpr  CylinderLengthUnits=cm  SphereRadius=1  SphereRadiusUnits=m  EllipsoidRadii=[1 1 1]  EllipsoidRadiiUnits=m  ExtrusionCrossSection=[1 1; -1 1; -1 -1; 1 -1]  ExtrusionCrossSectionUnits=m  ExtrusionLength=1  ExtrusionLengthUnits=m  PolygonNumSides=3  PolygonOuterRadius=1  PolygonOuterRadiusUnits=m  ExtGeomFileType=STL  ExtGeomFileUnits=m  RevolutionCrossSection=[1 1; 1 -1; 2 -1; 2 1]  RevolutionCrossSectionUnits=m  RevolutionExtent=Full  RevolutionAngle=180  RevolutionAngleUnits=deg  BlockFunction=simmechanics.library.body_elements.solid
  B : PMIOPort  Port=1  Side=Right
  H : PMIOPort  Port=2  Side=Left
  connections:
  H/RConn1 -- Bracket/RConn1
  Flange Transform/RConn1 -- Bracket/LConn1
  Piston Rod/RConn1 -- Flange Transform/LConn1 -- Base Transform/LConn1
  B/RConn1 -- Piston Head/RConn1 -- Base Transform/RConn1

== system wing_landing_gear/Wing Landing Gear/Main Column/Main Column/Art Links Bracket Housing ==
  Annular Cylinder : sm_wing_landing_gear_lib/Annular Cylinder  Ro=Ro  Ri=Ri  L=L  rho=rho  clr=clr  opc=1
  Left Side Transform : sm_lib/Frames and Transforms/Rigid Transform  TranslationMethod=Cylindrical  TranslationLengthUnit=cm  TranslationStandardAxis=-Y  TranslationStandardOffset=0  TranslationCartesianOffset=[0 0 0]  TranslationROffset=Ro  TranslationROffsetUnits=cm  TranslationZOffset=L/2  TranslationZOffsetUnits=cm  TranslationThetaOffset=-90  TranslationThetaOffsetUnits=deg  RotationMethod=AlignedAxes  RotationAngleUnits=deg  RotationStandardAxis=+Z  RotationAngle=0  RotationArbitraryAxis=[0 0 1]  FollAlignAxisA=+X  BaseAlignAxisA=-Y  FollAlignAxisB=+Y  BaseAlignAxisB=+X  RotationMatrix=[1 0 0; 0 1 0; 0 0 1]  BlockFunction=simmechanics.library.frames_transforms.rigid_transform
  Right Side Transform : sm_lib/Frames and Transforms/Rigid Transform  TranslationMethod=Cylindrical  TranslationLengthUnit=cm  TranslationStandardAxis=-Y  TranslationStandardOffset=0  TranslationCartesianOffset=[0 0 0]  TranslationROffset=Ro  TranslationROffsetUnits=cm  TranslationZOffset=L/2  TranslationZOffsetUnits=cm  TranslationThetaOffset=90  TranslationThetaOffsetUnits=deg  RotationMethod=AlignedAxes  RotationAngleUnits=deg  RotationStandardAxis=+Z  RotationAngle=0  RotationArbitraryAxis=[0 0 1]  FollAlignAxisA=+X  BaseAlignAxisA=+Y  FollAlignAxisB=+Y  BaseAlignAxisB=-X  RotationMatrix=[1 0 0; 0 1 0; 0 0 1]  BlockFunction=simmechanics.library.frames_transforms.rigid_transform
  T : PMIOPort  Port=1  Side=Right
  L : PMIOPort  Port=2  Side=Left
  B : PMIOPort  Port=3  Side=Left
  R : PMIOPort  Port=4  Side=Left
  connections:
  Left Side Transform/RConn1 -- L/RConn1
  T/RConn1 -- Annular Cylinder/RConn1
  Right Side Transform/RConn1 -- R/RConn1
  Left Side Transform/LConn1 -- Right Side Transform/LConn1 -- Annular Cylinder/LConn1 -- B/RConn1

== system wing_landing_gear/Wing Landing Gear/Main Column/Main Column/Main Actuator Bracket Housing ==
  Annular Cylinder : sm_wing_landing_gear_lib/Annular Cylinder  Ro=Ro  Ri=Ri  L=L  rho=rho  clr=clr  opc=1
  Left Side Transform : sm_lib/Frames and Transforms/Rigid Transform  TranslationMethod=Cylindrical  TranslationLengthUnit=cm  TranslationStandardAxis=-Y  TranslationStandardOffset=0  TranslationCartesianOffset=[0 0 0]  TranslationROffset=Ro  TranslationROffsetUnits=cm  TranslationZOffset=L/2  TranslationZOffsetUnits=cm  TranslationThetaOffset=180  TranslationThetaOffsetUnits=deg  RotationMethod=AlignedAxes  RotationAngleUnits=deg  RotationStandardAxis=+Z  RotationAngle=0  RotationArbitraryAxis=[0 0 1]  FollAlignAxisA=+X  BaseAlignAxisA=-X  FollAlignAxisB=+Y  BaseAlignAxisB=-Y  RotationMatrix=[1 0 0; 0 1 0; 0 0 1]  BlockFunction=simmechanics.library.frames_transforms.rigid_transform
  Right Side Transform : sm_lib/Frames and Transforms/Rigid Transform  TranslationMethod=Cylindrical  TranslationLengthUnit=cm  TranslationStandardAxis=-Y  TranslationStandardOffset=0  TranslationCartesianOffset=[0 0 0]  TranslationROffset=Ro  TranslationROffsetUnits=cm  TranslationZOffset=L/2  TranslationZOffsetUnits=cm  TranslationThetaOffset=0  TranslationThetaOffsetUnits=deg  RotationMethod=None  RotationAngleUnits=deg  RotationStandardAxis=+Z  RotationAngle=0  RotationArbitraryAxis=[0 0 1]  FollAlignAxisA=+X  BaseAlignAxisA=+Y  FollAlignAxisB=+Y  BaseAlignAxisB=-X  RotationMatrix=[1 0 0; 0 1 0; 0 0 1]  BlockFunction=simmechanics.library.frames_transforms.rigid_transform
  T : PMIOPort  Port=1  Side=Right
  L : PMIOPort  Port=2  Side=Left
  B : PMIOPort  Port=3  Side=Left
  R : PMIOPort  Port=4  Side=Left
  connections:
  B/RConn1 -- Annular Cylinder/LConn1 -- Right Side Transform/LConn1 -- Left Side Transform/LConn1
  Right Side Transform/RConn1 -- R/RConn1
  T/RConn1 -- Annular Cylinder/RConn1
  Left Side Transform/RConn1 -- L/RConn1

== system wing_landing_gear/Wing Landing Gear/Main Column/Main Column/Main Column Bottom Cylinder ==
  Annular Cylinder : sm_wing_landing_gear_lib/Annular Cylinder  Ro=Ro  Ri=Ri  L=L  rho=rho  clr=clr  opc=1
  Side Transform : sm_lib/Frames and Transforms/Rigid Transform  TranslationMethod=Cylindrical  TranslationLengthUnit=cm  TranslationStandardAxis=+X  TranslationStandardOffset=0  TranslationCartesianOffset=[ 0 0]  TranslationROffset=Ro  TranslationROffsetUnits=cm  TranslationZOffset=Oh  TranslationZOffsetUnits=cm  TranslationThetaOffset=Ah  TranslationThetaOffsetUnits=deg  RotationMethod=StandardAxis  RotationAngleUnits=deg  RotationStandardAxis=+Z  RotationAngle=Ah  RotationArbitraryAxis=[0 0 1]  FollAlignAxisA=+X  BaseAlignAxisA=+Y  FollAlignAxisB=+Y  BaseAlignAxisB=+Z  RotationMatrix=[1 0 0; 0 1 0; 0 0 1]  BlockFunction=simmechanics.library.frames_transforms.rigid_transform
  B : PMIOPort  Port=1  Side=Left
  T : PMIOPort  Port=2  Side=Right
  D : PMIOPort  Port=3  Side=Left
  connections:
  Side Transform/LConn1 -- Annular Cylinder/LConn1 -- B/RConn1
  Annular Cylinder/RConn1 -- T/RConn1
  Side Transform/RConn1 -- D/RConn1

== system wing_landing_gear/Wing Landing Gear/Main Column/Main Column/Main Column Top Cylinder ==
  Annular Cylinder : sm_wing_landing_gear_lib/Annular Cylinder  Ro=Ro  Ri=Ri  L=L  rho=rho  clr=clr  opc=1
  B : PMIOPort  Port=1  Side=Left
  T : PMIOPort  Port=2  Side=Right
  connections:
  Annular Cylinder/RConn1 -- T/RConn1
  B/RConn1 -- Annular Cylinder/LConn1

== system wing_landing_gear/Wing Landing Gear/Main Column/Main Column/Piston  ==
  Flange : sm_wing_landing_gear_lib/Annular Cylinder  Ro=Rf  Ri=Ri  L=Tf  rho=rho_alum  clr=clr  opc=1
  Piston : sm_wing_landing_gear_lib/Annular Cylinder  Ro=Ro  Ri=Ri  L=L  rho=rho_alum  clr=clr  opc=1
  B : PMIOPort  Port=1  Side=Right
  T : PMIOPort  Port=2  Side=Left
  connections:
  B/RConn1 -- Flange/LConn1
  Piston/RConn1 -- T/RConn1
  Flange/RConn1 -- Piston/LConn1

== system wing_landing_gear/Wing Landing Gear/Main Column/Main Column/Spherical Cup and Holder ==
  Cup : Subsystem  mask{Rb=Rci, Ro=Rco, T=2, A=210, Cc=cclr}
      mask prompts: Rb "Ball radius:"; Ro "Cup outer radius:"; T "Strip thickness:"; A "Cup angle:"; Cc "Color:"
      mask init:
      | theta = (linspace(-(A/2+90),(A/2-90),A+1)*pi/180)';
      | cup_profile = [Ro*cos(theta) Ro*sin(theta)];
      | theta = (linspace((A/2-90),-(A/2+90),A+1)*pi/180)';
      | cup_profile = vertcat(cup_profile,[Rb*cos(theta) Rb*sin(theta)]);
  Holder Half A : sm_lib/Body Elements/Solid  InertiaType=CalculateFromGeometry  Mass=1  MassUnits=kg  CenterOfMass=[0 0 0]  CenterOfMassUnits=m  MomentsOfInertia=[1 1 1]  MomentsOfInertiaUnits=kg*m^2  ProductsOfInertia=[0 0 0]  ProductsOfInertiaUnits=kg*m^2  DensityBased=on  Density=rho  DensityUnits=kg/(m^3)  GraphicType=FromGeometry  MarkerShape=Sphere  MarkerSize=10  MarkerSizeUnits=m  GraphicVisPropType=SimpleVisualProperties  GraphicDiffuseColor=hclr  GraphicSpecularColor=[0.5 0.5 0.5 1.0]  GraphicAmbientColor=[0.5 0.0 0.0 1.0]  GraphicEmissiveColor=[0.0 0.0 0.0 1.0]  GraphicShininess=75  GraphicOpacity=1.0  GeometryShape=GeneralExtrusion  RectangleSize=[1 1]  RectangleSizeUnits=m  BrickDimensions=[1 1 1]  BrickDimensionUnits=m  CylinderRadius=1  CylinderRadiusUnits=m  CylinderLength=1  CylinderLengthUnits=m  SphereRadius=1  SphereRadiusUnits=m  EllipsoidRadii=[1 1 1]  EllipsoidRadiiUnits=m  ExtrusionCrossSection=hinge_sec_a  ExtrusionCrossSectionUnits=cm  ExtrusionLength=Hh  ExtrusionLengthUnits=cm  PolygonNumSides=3  PolygonOuterRadius=1  PolygonOuterRadiusUnits=m  ExtGeomFileType=STL  ExtGeomFileUnits=m  RevolutionCrossSection=[1 1; 1 -1; 2 -1; 2 1]  RevolutionCrossSectionUnits=m  RevolutionExtent=Full  RevolutionAngle=180  RevolutionAngleUnits=deg  BlockFunction=simmechanics.library.body_elements.solid
  Holder Half B : sm_lib/Body Elements/Solid  InertiaType=CalculateFromGeometry  Mass=1  MassUnits=kg  CenterOfMass=[0 0 0]  CenterOfMassUnits=m  MomentsOfInertia=[1 1 1]  MomentsOfInertiaUnits=kg*m^2  ProductsOfInertia=[0 0 0]  ProductsOfInertiaUnits=kg*m^2  DensityBased=on  Density=rho  DensityUnits=kg/(m^3)  GraphicType=FromGeometry  MarkerShape=Sphere  MarkerSize=10  MarkerSizeUnits=m  GraphicVisPropType=SimpleVisualProperties  GraphicDiffuseColor=hclr  GraphicSpecularColor=[0.5 0.5 0.5 1.0]  GraphicAmbientColor=[0.5 0.0 0.0 1.0]  GraphicEmissiveColor=[0.0 0.0 0.0 1.0]  GraphicShininess=75  GraphicOpacity=1.0  GeometryShape=GeneralExtrusion  RectangleSize=[1 1]  RectangleSizeUnits=m  BrickDimensions=[1 1 1]  BrickDimensionUnits=m  CylinderRadius=1  CylinderRadiusUnits=m  CylinderLength=1  CylinderLengthUnits=m  SphereRadius=1  SphereRadiusUnits=m  EllipsoidRadii=[1 1 1]  EllipsoidRadiiUnits=m  ExtrusionCrossSection=hinge_sec_b  ExtrusionCrossSectionUnits=cm  ExtrusionLength=Hh  ExtrusionLengthUnits=cm  PolygonNumSides=3  PolygonOuterRadius=1  PolygonOuterRadiusUnits=m  ExtGeomFileType=STL  ExtGeomFileUnits=m  RevolutionCrossSection=[1 1; 1 -1; 2 -1; 2 1]  RevolutionCrossSectionUnits=m  RevolutionExtent=Full  RevolutionAngle=180  RevolutionAngleUnits=deg  BlockFunction=simmechanics.library.body_elements.solid
  Holder-Cup Transform : sm_lib/Frames and Transforms/Rigid Transform  TranslationMethod=Cartesian  TranslationLengthUnit=cm  TranslationStandardAxis=+X  TranslationStandardOffset=0  TranslationCartesianOffset=[Oh 0 Hh/2]  TranslationROffset=0  TranslationROffsetUnits=m  TranslationZOffset=0  TranslationZOffsetUnits=m  TranslationThetaOffset=0  TranslationThetaOffsetUnits=deg  RotationMethod=None  RotationAngleUnits=deg  RotationStandardAxis=+Z  RotationAngle=0  RotationArbitraryAxis=[0 0 1]  FollAlignAxisA=+X  BaseAlignAxisA=+Y  FollAlignAxisB=+Y  BaseAlignAxisB=+Z  RotationMatrix=[1 0 0; 0 1 0; 0 0 1]  BlockFunction=simmechanics.library.frames_transforms.rigid_transform
  S : PMIOPort  Port=1  Side=Right
  B : PMIOPort  Port=2  Side=Left
  connections:
  B/RConn1 -- Holder Half A/RConn1 -- Holder-Cup Transform/LConn1 -- Holder Half B/RConn1
  Holder-Cup Transform/RConn1 -- Cup/LConn1
  Cup/RConn1 -- S/RConn1

== system wing_landing_gear/Wing Landing Gear/Main Column Locking Mechanism/Side Stay Linkage/Peg and Ball ==
  Ball : sm_lib/Body Elements/Solid  InertiaType=CalculateFromGeometry  Mass=1  MassUnits=kg  CenterOfMass=[0 0 0]  CenterOfMassUnits=m  MomentsOfInertia=[1 1 1]  MomentsOfInertiaUnits=kg*m^2  ProductsOfInertia=[0 0 0]  ProductsOfInertiaUnits=kg*m^2  DensityBased=on  Density=rho  DensityUnits=kg/(m^3)  GraphicType=FromGeometry  MarkerShape=Sphere  MarkerSize=10  MarkerSizeUnits=m  GraphicVisPropType=SimpleVisualProperties  GraphicDiffuseColor=clr  GraphicSpecularColor=[0.5 0.5 0.5 1.0]  GraphicAmbientColor=[0.5 0.0 0.0 1.0]  GraphicEmissiveColor=[0.0 0.0 0.0 1.0]  GraphicShininess=75  GraphicOpacity=1.0  GeometryShape=Sphere  RectangleSize=[1 1]  RectangleSizeUnits=m  BrickDimensions=[1 1 1]  BrickDimensionUnits=m  CylinderRadius=0  CylinderRadiusUnits=mm  CylinderLength=0  CylinderLengthUnits=mm  SphereRadius=Rb  SphereRadiusUnits=cm  EllipsoidRadii=[1 1 1]  EllipsoidRadiiUnits=m  ExtrusionCrossSection=[1 1; -1 1; -1 -1; 1 -1]  ExtrusionCrossSectionUnits=m  ExtrusionLength=1  ExtrusionLengthUnits=m  PolygonNumSides=3  PolygonOuterRadius=1  PolygonOuterRadiusUnits=m  ExtGeomFileType=STL  ExtGeomFileUnits=m  RevolutionCrossSection=[1 1; 1 -1; 2 -1; 2 1]  RevolutionCrossSectionUnits=m  RevolutionExtent=Full  RevolutionAngle=180  RevolutionAngleUnits=deg  BlockFunction=simmechanics.library.body_elements.solid
  Base-Peg Transform : sm_lib/Frames and Transforms/Rigid Transform  TranslationMethod=StandardAxis  TranslationLengthUnit=cm  TranslationStandardAxis=+Z  TranslationStandardOffset=Lp/2  TranslationCartesianOffset=[0 0 0]  TranslationROffset=0  TranslationROffsetUnits=m  TranslationZOffset=0  TranslationZOffsetUnits=m  TranslationThetaOffset=0  TranslationThetaOffsetUnits=deg  RotationMethod=None  RotationAngleUnits=deg  RotationStandardAxis=+Z  RotationAngle=0  RotationArbitraryAxis=[0 0 1]  FollAlignAxisA=+Z  BaseAlignAxisA=+X  FollAlignAxisB=+X  BaseAlignAxisB=-Z  RotationMatrix=[1 0 0; 0 1 0; 0 0 1]  BlockFunction=simmechanics.library.frames_transforms.rigid_transform
  Peg : sm_lib/Body Elements/Solid  InertiaType=CalculateFromGeometry  Mass=1  MassUnits=kg  CenterOfMass=[0 0 0]  CenterOfMassUnits=m  MomentsOfInertia=[1 1 1]  MomentsOfInertiaUnits=kg*m^2  ProductsOfInertia=[0 0 0]  ProductsOfInertiaUnits=kg*m^2  DensityBased=on  Density=rho  DensityUnits=kg/(m^3)  GraphicType=FromGeometry  MarkerShape=Sphere  MarkerSize=10  MarkerSizeUnits=m  GraphicVisPropType=SimpleVisualProperties  GraphicDiffuseColor=clr  GraphicSpecularColor=[0.5 0.5 0.5 1.0]  GraphicAmbientColor=[0.5 0.0 0.0 1.0]  GraphicEmissiveColor=[0.0 0.0 0.0 1.0]  GraphicShininess=75  GraphicOpacity=1.0  GeometryShape=Cylinder  RectangleSize=[1 1]  RectangleSizeUnits=m  BrickDimensions=[1 1 1]  BrickDimensionUnits=m  CylinderRadius=Rp  CylinderRadiusUnits=cm  CylinderLength=Lp  CylinderLengthUnits=cm  SphereRadius=1  SphereRadiusUnits=m  EllipsoidRadii=[1 1 1]  EllipsoidRadiiUnits=m  ExtrusionCrossSection=[1 1; -1 1; -1 -1; 1 -1]  ExtrusionCrossSectionUnits=m  ExtrusionLength=1  ExtrusionLengthUnits=m  PolygonNumSides=3  PolygonOuterRadius=1  PolygonOuterRadiusUnits=m  ExtGeomFileType=STL  ExtGeomFileUnits=m  RevolutionCrossSection=[1 1; 1 -1; 2 -1; 2 1]  RevolutionCrossSectionUnits=m  RevolutionExtent=Full  RevolutionAngle=180  RevolutionAngleUnits=deg  BlockFunction=simmechanics.library.body_elements.solid
  Peg-Ball Transform : sm_lib/Frames and Transforms/Rigid Transform  TranslationMethod=StandardAxis  TranslationLengthUnit=cm  TranslationStandardAxis=+Z  TranslationStandardOffset=Lp/2  TranslationCartesianOffset=[0 0 0]  TranslationROffset=0  TranslationROffsetUnits=m  TranslationZOffset=0  TranslationZOffsetUnits=m  TranslationThetaOffset=0  TranslationThetaOffsetUnits=deg  RotationMethod=None  RotationAngleUnits=deg  RotationStandardAxis=+Z  RotationAngle=0  RotationArbitraryAxis=[0 0 1]  FollAlignAxisA=+Z  BaseAlignAxisA=+X  FollAlignAxisB=+X  BaseAlignAxisB=-Z  RotationMatrix=[1 0 0; 0 1 0; 0 0 1]  BlockFunction=simmechanics.library.frames_transforms.rigid_transform
  F : PMIOPort  Port=1  Side=Right
  B : PMIOPort  Port=2  Side=Left
  connections:
  Base-Peg Transform/LConn1 -- B/RConn1
  Ball/RConn1 -- F/RConn1 -- Peg-Ball Transform/RConn1
  Base-Peg Transform/RConn1 -- Peg-Ball Transform/LConn1 -- Peg/RConn1
